simulink model "solver"  (R2018b)
settings: Solver=FixedStepDiscrete  StartTime=0.0  StopTime=1.0  FixedStep=0.1  MaxStep=0.1  RelTol=1e-3
libraries: simulink x2
settings Model: Creator=marwan  LastModifiedBy=marwan
settings DataIOCC: ExternalInput=[t,u]  LoadExternalInput=on

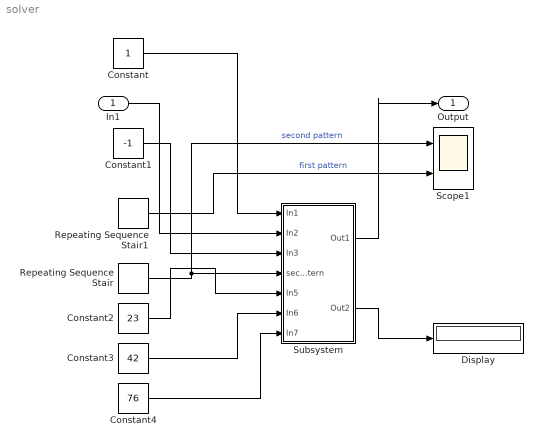
== system solver ==
  In1 : Inport
  Constant : Constant
  Constant1 : Constant  Value=-1
  Constant2 : Constant  Value=23
  Constant3 : Constant  Value=42
  Constant4 : Constant  Value=76
  Display : Display
  Repeating Sequence Stair : simulink/Sources/Repeating Sequence Stair  OutValues=[1 3 2 3 1 2]  tsamp=-1  OutMin=[]  OutMax=[]  OutDataTypeStr=double  OutputDataTypeScalingMode=double  OutDataType=fixdt(0,8)  ConRadixGroup=Best Precision: Vector-wise  OutScaling=2^-12
  Repeating Sequence Stair1 : simulink/Sources/Repeating Sequence Stair  OutValues=[12 3 12 3 14 2]  tsamp=-1  OutMin=[]  OutMax=[]  OutDataTypeStr=double  OutputDataTypeScalingMode=double  OutDataType=fixdt(0,8)  ConRadixGroup=Best Precision: Vector-wise  OutScaling=2^-12
  Scope1 : Scope  NumInputPorts=2
  Subsystem : Subsystem  TreatAsAtomicUnit=on
  Output : Outport
  wires:
  Repeating Sequence Stair/1 -> Scope1/1, Subsystem/4(second pattern)  "second pattern"
  Repeating Sequence Stair1/1 -> Scope1/2  "first pattern"
  Constant/1 -> Subsystem/1(In1)
  In1/1 -> Subsystem/2(In2)
  Constant1/1 -> Subsystem/3(In3)
  Constant2/1 -> Subsystem/5(In5)
  Constant3/1 -> Subsystem/6(In6)
  Constant4/1 -> Subsystem/7(In7)
  Subsystem/1(Out1) -> Output/1
  Subsystem/2(Out2) -> Display/1

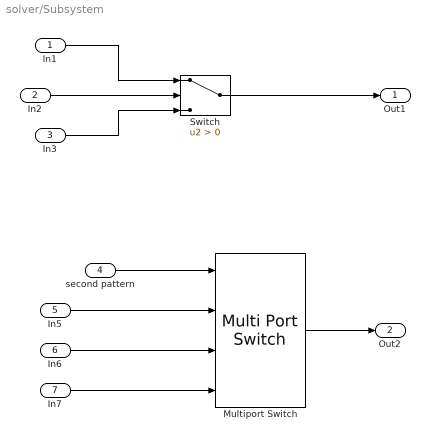
== system solver/Subsystem ==
  In1 : Inport
  In2 : Inport  Port=2
  In3 : Inport  Port=3
  second pattern : Inport  Port=4
  In5 : Inport  Port=5
  In6 : Inport  Port=6
  In7 : Inport  Port=7
  Multiport Switch : MultiPortSwitch
  Switch : Switch  Criteria=u2 > Threshold
  Out1 : Outport
  Out2 : Outport  Port=2
  wires:
  In2/1 -> Switch/2
  Switch/1 -> Out1/1
  In3/1 -> Switch/3
  second pattern/1 -> Multiport Switch/1
  In1/1 -> Switch/1
  Multiport Switch/1 -> Out2/1
  In7/1 -> Multiport Switch/4
  In6/1 -> Multiport Switch/3
  In5/1 -> Multiport Switch/2
